simulink model "Hodgkin-Huxely_models"  (R2017a)
settings: Solver=ode1  StartTime=0.0  StopTime=10  FixedStep=0.001  RelTol=1e-3  EnableMultiTasking=on
settings Model: Creator=MURAT  LastModifiedBy=Swapnil
settings DataIOCC: LimitDataPoints=on  SaveFormat=Array  SignalLoggingSaveFormat=ModelDataLogs
settings OptimizationCC: InitFltsAndDblsToZero=on  LifeSpan=inf
settings DebuggingCC: SaveWithParameterizedLinksMsg=none  UnderspecifiedInitializationDetection=Classic  MergeDetectMultiDrivingBlocksExec=none  SignalResolutionControl=TryResolveAllWithWarning  SolverPrmCheckMsg=warning  FcnCallInpInsideContextMsg=warning  SFUnexpectedBacktrackingDiag=warning  SFNoUnconditionalDefaultTransitionDiag=warning  SFExecutionAtInitializationDiag=none
settings HardwareCC: ProdBitPerPointer=32  ProdBitPerSizeT=32  ProdBitPerPtrDiffT=32  ProdLargestAtomicFloat=None  ProdIntDivRoundTo=Undefined  ProdEndianess=Unspecified  ProdWordSize=32  ProdHWDeviceType=32-bit Generic
settings ModelReferenceCC: PropagateSignalLabelsOutOfModel=off
settings GRTTargetCC: TargetFcnLib=ansi_tfl_tmw.mat  TargetLangStandard=C89/C90 (ANSI)  CombineOutputUpdateFcns=off  GRTInterface=on
settings ConfigComp: CovMetricSettings=dw  CovHtmlReporting=on  CovSaveCumulativeToWorkspaceVar=on  CovSaveSingleToWorkspaceVar=on  CovExternalEMLEnable=off

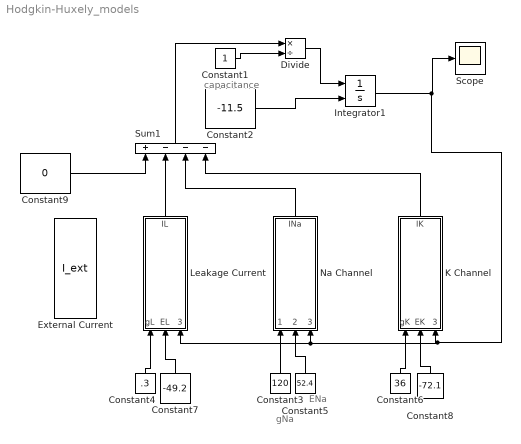
== system Hodgkin-Huxely_models ==
  note: ENa
  note: gNa
  note: capacitance
  Constant1 : Constant
  Constant2 : Constant  Value=-11.5
  Constant3 : Constant  Value=120
  Constant4 : Constant  Value=.3
  Constant5 : Constant  Value=52.4
  Constant6 : Constant  Value=36
  Constant7 : Constant  Value=-49.2
  Constant8 : Constant  Value=-72.1
  Constant9 : Constant  Value=0
  Divide : Product  Inputs=*/
  External Current : FromWorkspace  VariableName=I_ext  SampleTime=0
  Integrator1 : Integrator  InitialConditionSource=external
  K Channel : Subsystem
  Leakage Current : Subsystem
  Na Channel : Subsystem
  Scope : Scope
  Sum1 : Sum  Inputs=+---
  wires:
  Leakage Current/1(IL) -> Sum1/2
  Na Channel/1(INa) -> Sum1/3
  K Channel/1(IK) -> Sum1/4
  Constant2/1 -> Integrator1/2
  Constant3/1 -> Na Channel/1(gNa)
  Constant6/1 -> K Channel/1(gK)
  Constant4/1 -> Leakage Current/1(gL)
  Constant7/1 -> Leakage Current/2(EL)
  Constant5/1 -> Na Channel/2(ENa)
  Constant8/1 -> K Channel/2(EK)
  Integrator1/1 -> Leakage Current/3(vm), Na Channel/3(Vm), K Channel/3(vm), Scope/1
  Sum1/1 -> Divide/1
  Divide/1 -> Integrator1/1
  Constant1/1 -> Divide/2
  Constant9/1 -> Sum1/1

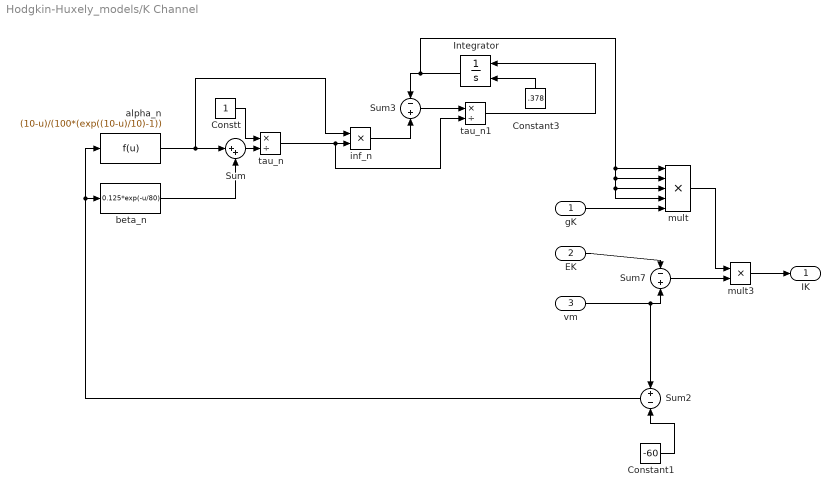
== system Hodgkin-Huxely_models/K Channel ==
  gK : Inport
  EK : Inport  Port=2
  vm : Inport  Port=3
  Constant1 : Constant  Value=-60
  Constant3 : Constant  Value=.378
  Constt : Constant
  Integrator : Integrator  InitialConditionSource=external
  Sum : Sum  Inputs=|++
  Sum2 : Sum  Inputs=+-
  Sum3 : Sum  Inputs=-+
  Sum7 : Sum  Inputs=-+
  alpha_n : Fcn  Expr=(10-u)/(100*(exp((10-u)/10)-1))
  beta_n : Fcn  Expr=0.125*exp(-u/80)
  inf_n : Product  Inputs=**
  mult : Product  Inputs=*****
  mult3 : Product  Inputs=**
  tau_n : Product  Inputs=*/
  tau_n1 : Product  Inputs=*/
  IK : Outport
  wires:
  mult3/1 -> IK/1
  vm/1 -> Sum2/1, Sum7/2
  EK/1 -> Sum7/1
  gK/1 -> mult/5
  Sum7/1 -> mult3/2
  mult/1 -> mult3/1
  Constant3/1 -> Integrator/2
  tau_n1/1 -> Integrator/1
  Sum3/1 -> tau_n1/1
  inf_n/1 -> Sum3/2
  Integrator/1 -> Sum3/1, mult/1, mult/2, mult/3, mult/4
  tau_n/1 -> inf_n/2, tau_n1/2
  Sum/1 -> tau_n/2
  Constt/1 -> tau_n/1
  beta_n/1 -> Sum/2
  alpha_n/1 -> Sum/1, inf_n/1
  Constant1/1 -> Sum2/2
  Sum2/1 -> alpha_n/1, beta_n/1

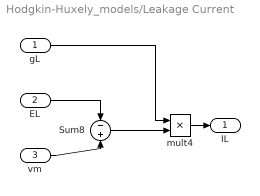
== system Hodgkin-Huxely_models/Leakage Current ==
  gL : Inport
  EL : Inport  Port=2
  vm : Inport  Port=3
  Sum8 : Sum  Inputs=-+
  mult4 : Product  Inputs=**
  IL : Outport
  wires:
  Sum8/1 -> mult4/2
  gL/1 -> mult4/1
  EL/1 -> Sum8/1
  vm/1 -> Sum8/2
  mult4/1 -> IL/1

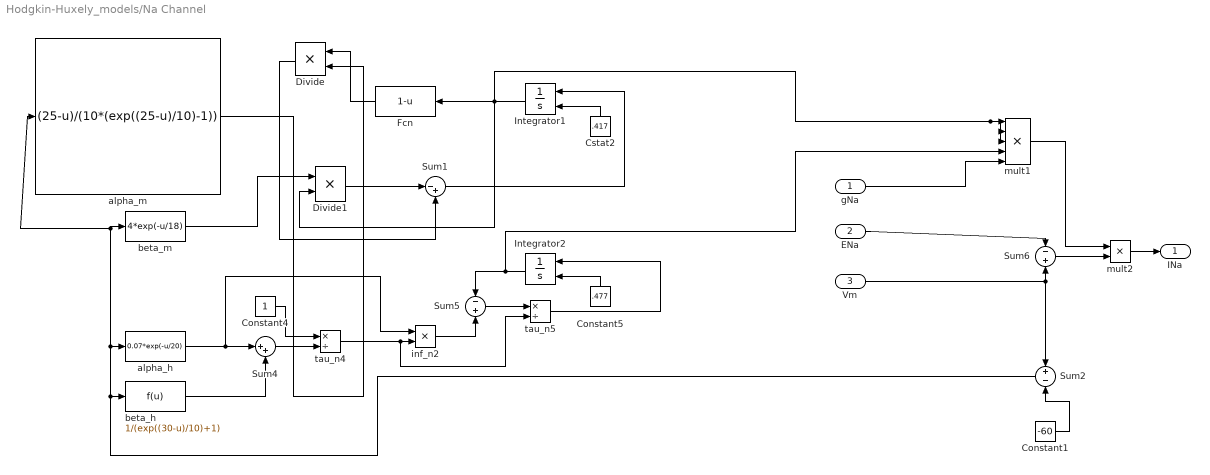
== system Hodgkin-Huxely_models/Na Channel ==
  gNa : Inport
  ENa : Inport  Port=2
  Vm : Inport  Port=3
  Constant1 : Constant  Value=-60
  Constant4 : Constant
  Constant5 : Constant  Value=.477
  Cstat2 : Constant  Value=.417
  Divide : Product  Inputs=**
  Divide1 : Product  Inputs=**
  Fcn : Fcn  Expr=1-u
  Integrator1 : Integrator  InitialConditionSource=external
  Integrator2 : Integrator  InitialConditionSource=external
  Sum1 : Sum  Inputs=|-+
  Sum2 : Sum  Inputs=+-
  Sum4 : Sum  Inputs=|++
  Sum5 : Sum  Inputs=-+
  Sum6 : Sum  Inputs=-+
  alpha_h : Fcn  Expr=0.07*exp(-u/20)
  alpha_m : Fcn  Expr=(25-u)/(10*(exp((25-u)/10)-1))
  beta_h : Fcn  Expr=1/(exp((30-u)/10)+1)
  beta_m : Fcn  Expr=4*exp(-u/18)
  inf_n2 : Product  Inputs=**
  mult1 : Product  Inputs=*****
  mult2 : Product  Inputs=**
  tau_n4 : Product  Inputs=*/
  tau_n5 : Product  Inputs=*/
  INa : Outport
  wires:
  alpha_h/1 -> Sum4/1, inf_n2/1
  beta_h/1 -> Sum4/2
  Constant4/1 -> tau_n4/1
  Sum4/1 -> tau_n4/2
  Integrator1/1 -> Divide1/2, Fcn/1, mult1/2, mult1/3, mult1/1
  tau_n4/1 -> inf_n2/2, tau_n5/2
  Integrator2/1 -> Sum5/1, mult1/4
  inf_n2/1 -> Sum5/2
  Sum5/1 -> tau_n5/1
  tau_n5/1 -> Integrator2/1
  Constant5/1 -> Integrator2/2
  Sum1/1 -> Integrator1/1
  Cstat2/1 -> Integrator1/2
  Sum6/1 -> mult2/2
  gNa/1 -> mult1/5
  mult1/1 -> mult2/1
  ENa/1 -> Sum6/1
  Vm/1 -> Sum2/1, Sum6/2
  mult2/1 -> INa/1
  Fcn/1 -> Divide/1
  alpha_m/1 -> Divide/2
  beta_m/1 -> Divide1/1
  Divide1/1 -> Sum1/1
  Divide/1 -> Sum1/2
  Constant1/1 -> Sum2/2
  Sum2/1 -> alpha_m/1, beta_m/1, alpha_h/1, beta_h/1
